simulink model "11_2"  (R2018b)
settings: Solver=VariableStepAuto  StartTime=0.0  StopTime=5  MaxStep=0.01  RelTol=1e-3
values from neighbouring files (symbols this model uses):
  A = [0 1; 4 0]    [K_and_M_finder.m]    (also in Lf_and_Mf_finder.m; Output_Mf_Lf.m; solver.m)
  A_sh = [Gf zeros(2); Bf*Hf A]    [Mn_and_L_finder.m]
  B = [1; 1]    [K_and_M_finder.m]    (also in Lf_and_Mf_finder.m; Output_Mf_Lf.m; solver.m)
  B_sh = [zeros(2,1); B]    [Mn_and_L_finder.m]
  Bf = [2; 6]    [Lf_and_Mf_finder.m]    (also in Output_Mf_Lf.m; Output_Mf_sh.m)
  C = [3 0]    [Lf_and_Mf_finder.m]    (also in Output_Mf_Lf.m; solver.m)
  C_sh = [0 0 C]    [Mn_and_L_finder.m]    (also in Output_Mf_sh.m = [c1 c2])
  D = 3    [Lf_and_Mf_finder.m]    (also in Output_Mf_Lf.m; solver.m)
  Gf = [0 1; -9 0]    [Lf_and_Mf_finder.m]    (also in Mn_and_L_finder.m; Output_Mf_Lf.m; Output_Mf_sh.m)
  Hf = [1 0]    [Lf_and_Mf_finder.m]    (also in Mn_and_L_finder.m; Output_Mf_Lf.m; Output_Mf_sh.m)
  Kk = [k1Sol k2Sol]    [K_and_M_finder.m]
  L_sh = transpose(-Hn_sh * inv(Mn))    [Mn_and_L_finder.m]    (also in Output_Mf_sh.m = [0; 1]; solver.m = [0; 1])
  Lf = [l1Sol l2Sol]    [Lf_and_Mf_finder.m]
settings Model: Creator=kekos  LastModifiedBy=kekos

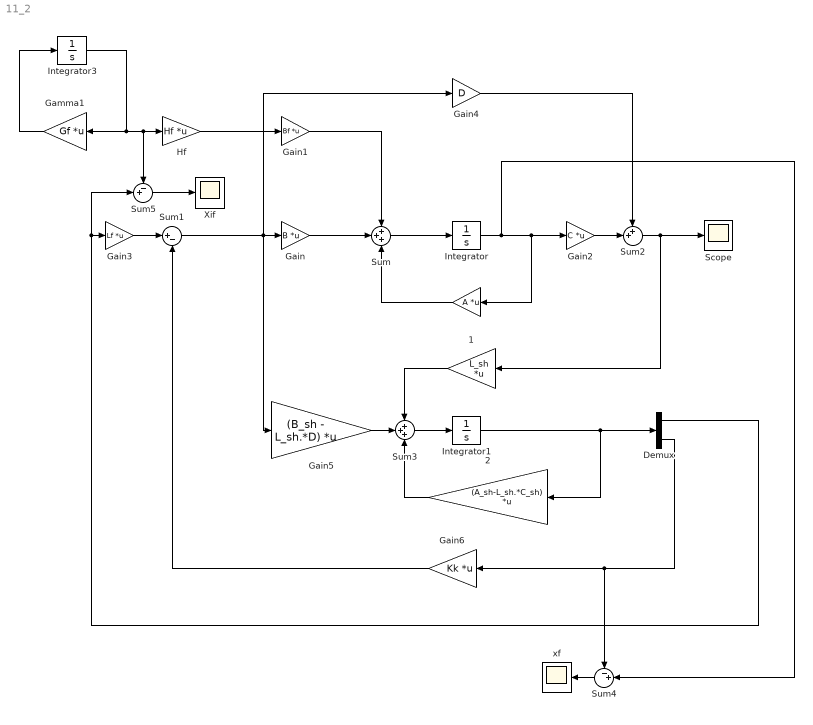
== system 11_2 ==
  " " : Gain  Gain=A  Multiplication=Matrix(K*u)
  " 1" : Gain  Gain=L_sh  Multiplication=Matrix(K*u)
  " 2" : Gain  Gain=(A_sh-L_sh.*C_sh)  Multiplication=Matrix(K*u)
  Demux : Demux  Outputs=2
  Gain : Gain  Gain=B  Multiplication=Matrix(K*u)
  Gain1 : Gain  Gain=Bf  Multiplication=Matrix(K*u)
  Gain2 : Gain  Gain=C  Multiplication=Matrix(K*u)
  Gain3 : Gain  Gain=Lf  Multiplication=Matrix(K*u)
  Gain4 : Gain  Gain=D
  Gain5 : Gain  Gain=(B_sh - L_sh.*D)  Multiplication=Matrix(K*u)
  Gain6 : Gain  Gain=Kk  Multiplication=Matrix(K*u)
  Gamma1 : Gain  Gain=Gf  Multiplication=Matrix(K*u)
  Hf : Gain  Gain=Hf  Multiplication=Matrix(K*u)
  Integrator : Integrator
  Integrator1 : Integrator  InitialCondition=[-2.91; -19.10; 0; 0]
  Integrator3 : Integrator  InitialCondition=[-2.91; -19.10]
  Scope : Scope
  Sum : Sum  Inputs=+++
  Sum1 : Sum  Inputs=|+-
  Sum2 : Sum  Inputs=++|
  Sum3 : Sum  Inputs=+++
  Sum4 : Sum  Inputs=-+|
  Sum5 : Sum  Inputs=-+|
  Xif : Scope
  xf : Scope
  wires:
  Gain4/1 -> Sum2/1
  Gain5/1 -> Sum3/2
  Sum3/1 -> Integrator1/1
  " 1"/1 -> Sum3/1
  " 2"/1 -> Sum3/3
  Sum2/1 -> " 1"/1, Scope/1
  Sum1/1 -> Gain5/1, Gain4/1, Gain/1
  Demux/1 -> Sum5/2, Gain3/1
  Gain2/1 -> Sum2/2
  Integrator/1 -> Sum4/2, Gain2/1, " "/1
  Integrator1/1 -> Demux/1, " 2"/1
  Sum/1 -> Integrator/1
  " "/1 -> Sum/3
  Gain/1 -> Sum/2
  Gain3/1 -> Sum1/1
  Demux/2 -> Gain6/1, Sum4/1
  Gain6/1 -> Sum1/2
  Hf/1 -> Gain1/1
  Gain1/1 -> Sum/1
  Sum4/1 -> xf/1
  Integrator3/1 -> Hf/1, Sum5/1, Gamma1/1
  Gamma1/1 -> Integrator3/1
  Sum5/1 -> Xif/1
